simulink model "MARC_Hinf"  (R2016b)
settings: Solver=VariableStepAuto  StartTime=0.0  StopTime=150  RelTol=1e-3
values from neighbouring files (symbols this model uses):
  Aa = [zeros(n,n) Cp;zeros(np,n) Ap]    [g_MRAC_design_Hinf.m]
  Aref = Aa - Ba*KxT    [g_MRAC_design_Hinf.m]
  Ba = [Dp;Bp]    [g_MRAC_design_Hinf.m]
  Bref = [-eye(n);zeros(np,n)]    [g_MRAC_design_Hinf.m]
  Ca = [zeros(n,n) Cp]    [g_MRAC_design_Hinf.m]
  Cref = Ca    [g_MRAC_design_Hinf.m]
  DA = 0.75*eye(n)    [g_MRAC_design_Hinf.m]
  Gama_theta_ = eye(13)*5    [g_MRAC_design_Hinf.m]
  if_sat_modification = 1    [g_MRAC_design_Hinf.m]
  KxT = [KI KF]    [g_Hinf_design.m]
  Lv = Pv*inv(Rv)    [g_MRAC_design_Hinf.m]
  Pv = are(Aref',inv(Rv), Qv)    [g_MRAC_design_Hinf.m]
undefined symbols (not defined in the file): n, np
libraries: simulink x10
settings Model: Creator=user  LastModifiedBy=xiaoliang

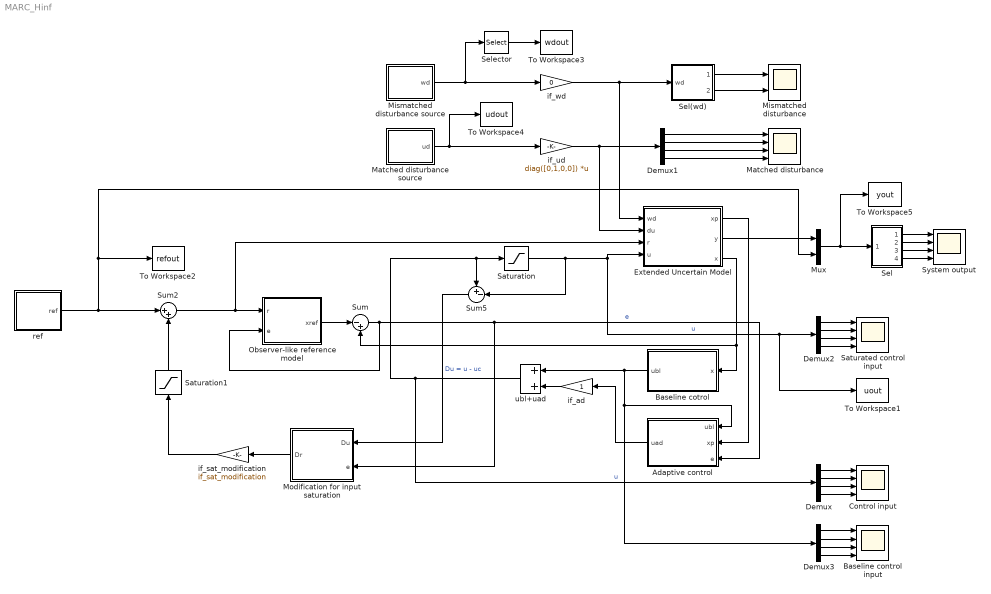
== system MARC_Hinf ==
  Adaptive control : Subsystem  mask{Gama_theta_=Gama_theta_, Pref=Pv, Ba=Ba, theta_max=[1 1 1 1.5]*1, es=[0.8 0.8 0.8 0.8]}
  Baseline control input : Scope  NumInputPorts=4
  Baseline cotrol : Subsystem  mask{KxT=KxT}
  Control input : Scope  NumInputPorts=4
  Demux{,1..3} (4 alike) : Demux
  Extended Uncertain Model : Subsystem  mask{Aa=Aa, Ba=Ba, Ca=Ca, Bref=Bref, Dex=[n+1:n+np], DA=DA, THETA0=rand(4,9)*0.5}
  Matched disturbance : Scope  NumInputPorts=4
  Matched disturbance source : Subsystem  mask{wb=0.2, k=0.5, Ts=0.001}
      mask prompts: wb "wb (Filter bandwidth)"; k "k (Signal standard deviation)"; Ts "Ts (Sample time)"
  Mismatched disturbance : Scope  NumInputPorts=2
  Mismatched disturbance source : Subsystem  mask{wb=2.5, k=0.4, Ts=0.001}
      mask prompts: wb "wb (Filter bandwidth)"; k "k (Signal standard deviation)"; Ts "Ts (Sample time)"
  Modification for input saturation : Subsystem  mask{Pv=Pv, Bref=Bref, Gama_du=-diag([1 1 1 1])*2}
  Mux : Mux  Inputs=2
  Observer-like reference model : Subsystem  mask{Aref=Aref, Bref=Bref, Cref=Cref, Lv=Lv}
  Saturated control input : Scope  NumInputPorts=4
  Saturation : Saturate  UpperLimit=inf  LowerLimit=-inf
  Saturation1 : Saturate  UpperLimit=1  LowerLimit=-1
  Sel : Subsystem
  Sel(wd) : Subsystem
  Selector : Selector  InputPortWidth=13  IndexOptions=Index vector (dialog)  Indices=[5:10]  OutputSizes=1
  Sum : Sum  Inputs=|-+
  Sum2 : Sum  Inputs=|++
  Sum5 : Sum  Inputs=+-|
  System output : Scope  NumInputPorts=4
  To Workspace1 : ToWorkspace  VariableName=uout  SaveFormat=Timeseries  SampleTime=-1
  To Workspace2 : ToWorkspace  VariableName=refout  SaveFormat=Timeseries  SampleTime=-1
  To Workspace3 : ToWorkspace  VariableName=wdout  SaveFormat=Timeseries  SampleTime=-1
  To Workspace4 : ToWorkspace  VariableName=udout  SaveFormat=Timeseries  SampleTime=-1
  To Workspace5 : ToWorkspace  VariableName=yout  SaveFormat=Timeseries  SampleTime=-1
  if_ad : Gain
  if_sat_modification : Gain  Gain=if_sat_modification
  if_ud : Gain  Gain=diag([0,1,0,0])  Multiplication=Matrix(K*u)
  if_wd : Gain  Gain=0
  ref : Subsystem
  ubl+uad : Sum
  wires:
  Mismatched disturbance source/1(wd) -> if_wd/1, Selector/1
  Extended Uncertain Model/3(x) -> Sum/2, Baseline cotrol/1(x)
  Extended Uncertain Model/1(xp) -> Adaptive control/2(xp)
  Observer-like reference model/1(xref) -> Sum/1
  Sum/1 -> Modification for input saturation/2(e), Adaptive control/3(e), Observer-like reference model/2(e)  "e"
  Adaptive control/1(uad) -> if_ad/1
  Baseline cotrol/1(ubl) -> Demux3/1, Adaptive control/1(ubl), ubl+uad/1
  Extended Uncertain Model/2(y) -> Mux/1
  Mux/1 -> Sel/1("[y;r]"), To Workspace5/1
  Sel/1(1) -> System output/1
  Sel/2(2) -> System output/2
  Sel/3(3) -> System output/3
  Sel/4(4) -> System output/4
  Matched disturbance source/1(ud) -> if_ud/1, To Workspace4/1
  ubl+uad/1 -> Saturation/1, Sum5/1, Demux/1  "u"
  Demux/1 -> Control input/1
  Demux/2 -> Control input/2
  Demux/3 -> Control input/3
  Demux/4 -> Control input/4
  if_wd/1 -> Extended Uncertain Model/1(wd), Sel(wd)/1(wd)
  if_ud/1 -> Demux1/1, Extended Uncertain Model/2(du)
  Demux1/1 -> Matched disturbance/1
  Demux1/2 -> Matched disturbance/2
  Demux1/3 -> Matched disturbance/3
  Demux1/4 -> Matched disturbance/4
  if_ad/1 -> ubl+uad/2
  Selector/1 -> To Workspace3/1
  Demux2/1 -> Saturated control input/1
  Demux2/2 -> Saturated control input/2
  Demux2/3 -> Saturated control input/3
  Demux2/4 -> Saturated control input/4
  Saturation/1 -> Sum5/2, To Workspace1/1, Demux2/1, Extended Uncertain Model/4(u)  "u"
  Sum2/1 -> Extended Uncertain Model/3(r), Observer-like reference model/1(r)
  ref/1(ref) -> Mux/2, To Workspace2/1, Sum2/1
  Modification for input saturation/1(Dr) -> if_sat_modification/1
  Sum5/1 -> Modification for input saturation/1(Du)  "Du = u - uc"
  if_sat_modification/1 -> Saturation1/1
  Sel(wd)/1(wd(1,2,3)) -> Mismatched disturbance/1
  Sel(wd)/2(wd(4,5,6)) -> Mismatched disturbance/2
  Saturation1/1 -> Sum2/2
  Demux3/1 -> Baseline control input/1
  Demux3/2 -> Baseline control input/2
  Demux3/3 -> Baseline control input/3
  Demux3/4 -> Baseline control input/4

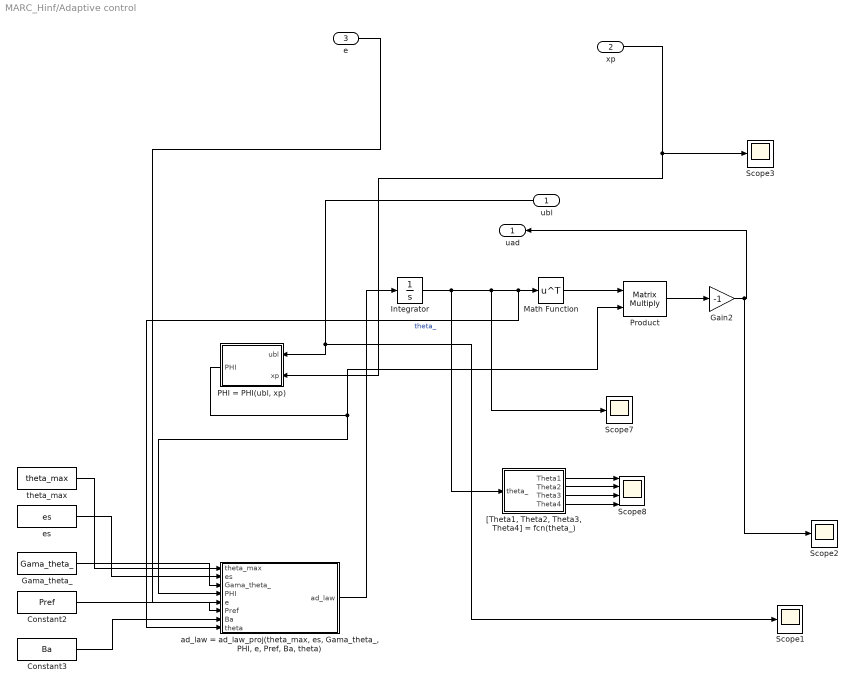
== system MARC_Hinf/Adaptive control ==
  ubl : Inport
  xp : Inport  Port=2
  e : Inport  Port=3
  Constant2 : Constant  Value=Pref
  Constant3 : Constant  Value=Ba
  Gain2 : Gain  Gain=-1
  Gama_theta_ : Constant  Value=Gama_theta_
  Integrator : Integrator  UpperSaturationLimit=4  LowerSaturationLimit=-4  IgnoreLimit=on
  Math Function : Math  Operator=transpose  SaturateOnIntegerOverflow=on
  "PHI = PHI(ubl, xp)" : MATLAB Function  TreatAsAtomicUnit=on
  Product : Product  Multiplication=Matrix(*)
  Scope{1..3,7} (4 alike) : Scope
  Scope8 : Scope  NumInputPorts=4
  "[Theta1, Theta2, Theta3, Theta4] = fcn(theta_)" : MATLAB Function  TreatAsAtomicUnit=on
  "ad_law = ad_law_proj(theta_max, es, Gama_theta_, PHI, e, Pref, Ba, theta)" : MATLAB Function  TreatAsAtomicUnit=on
  es : Constant  Value=es
  theta_max : Constant  Value=theta_max
  uad : Outport
  wires:
  Constant2/1 -> "ad_law = ad_law_proj(theta_max, es, Gama_theta_, PHI, e, Pref, Ba, theta)"/6(Pref)
  "[Theta1, Theta2, Theta3, Theta4] = fcn(theta_)"/1(Theta1) -> Scope8/1
  "[Theta1, Theta2, Theta3, Theta4] = fcn(theta_)"/2(Theta2) -> Scope8/2
  Gain2/1 -> Scope2/1, uad/1
  Integrator/1 -> "[Theta1, Theta2, Theta3, Theta4] = fcn(theta_)"/1(theta_), Scope7/1, "ad_law = ad_law_proj(theta_max, es, Gama_theta_, PHI, e, Pref, Ba, theta)"/8(theta), Math Function/1  "theta_"
  Math Function/1 -> Product/1
  Product/1 -> Gain2/1
  "ad_law = ad_law_proj(theta_max, es, Gama_theta_, PHI, e, Pref, Ba, theta)"/1(ad_law) -> Integrator/1
  Gama_theta_/1 -> "ad_law = ad_law_proj(theta_max, es, Gama_theta_, PHI, e, Pref, Ba, theta)"/3(Gama_theta_)
  e/1 -> "ad_law = ad_law_proj(theta_max, es, Gama_theta_, PHI, e, Pref, Ba, theta)"/5(e)
  "PHI = PHI(ubl, xp)"/1(PHI) -> "ad_law = ad_law_proj(theta_max, es, Gama_theta_, PHI, e, Pref, Ba, theta)"/4(PHI), Product/2
  Constant3/1 -> "ad_law = ad_law_proj(theta_max, es, Gama_theta_, PHI, e, Pref, Ba, theta)"/7(Ba)
  xp/1 -> Scope3/1, "PHI = PHI(ubl, xp)"/2(xp)
  ubl/1 -> Scope1/1, "PHI = PHI(ubl, xp)"/1(ubl)
  es/1 -> "ad_law = ad_law_proj(theta_max, es, Gama_theta_, PHI, e, Pref, Ba, theta)"/2(es)
  theta_max/1 -> "ad_law = ad_law_proj(theta_max, es, Gama_theta_, PHI, e, Pref, Ba, theta)"/1(theta_max)
  "[Theta1, Theta2, Theta3, Theta4] = fcn(theta_)"/3(Theta3) -> Scope8/3
  "[Theta1, Theta2, Theta3, Theta4] = fcn(theta_)"/4(Theta4) -> Scope8/4

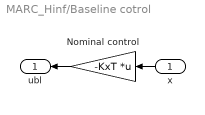
== system MARC_Hinf/Baseline cotrol ==
  x : Inport
  Nominal control : Gain  Gain=-KxT  Multiplication=Matrix(K*u)
  ubl : Outport
  wires:
  Nominal control/1 -> ubl/1
  x/1 -> Nominal control/1

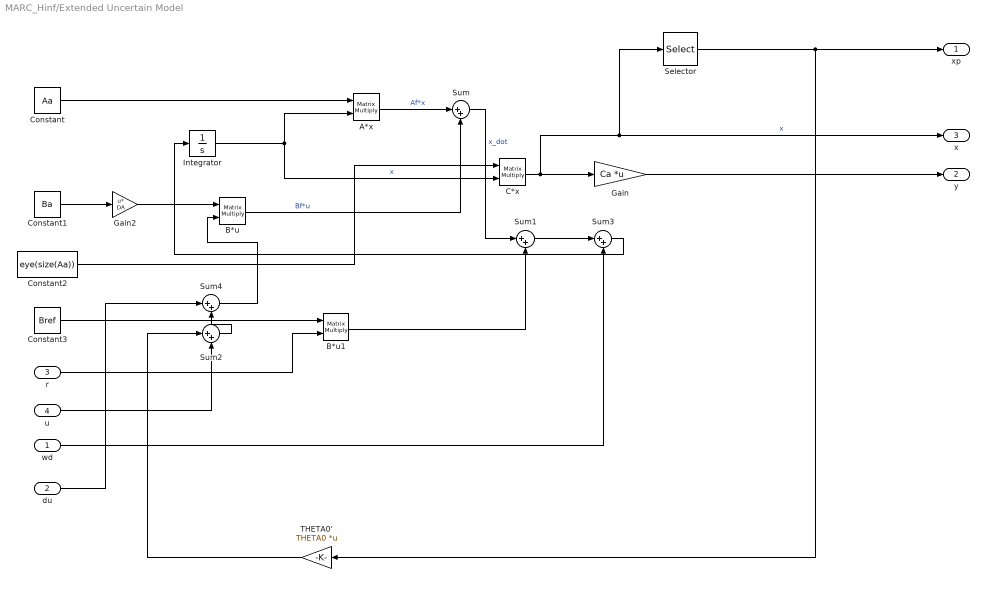
== system MARC_Hinf/Extended Uncertain Model ==
  wd : Inport
  du : Inport  Port=2
  r : Inport  Port=3
  u : Inport  Port=4
  A*x : Product  Multiplication=Matrix(*)
  B*u : Product  Multiplication=Matrix(*)
  B*u1 : Product  Multiplication=Matrix(*)
  C*x : Product  Multiplication=Matrix(*)
  Constant : Constant  Value=Aa
  Constant1 : Constant  Value=Ba
  Constant2 : Constant  Value=eye(size(Aa))
  Constant3 : Constant  Value=Bref
  Gain : Gain  Gain=Ca  Multiplication=Matrix(K*u)
  Gain2 : Gain  Gain=DA  Multiplication=Matrix(u*K)
  Integrator : Integrator  UpperSaturationLimit=1000  LowerSaturationLimit=-1000
  Selector : Selector  InputPortWidth=size(Aa,1)  IndexOptions=Index vector (dialog)  Indices=Dex  OutputSizes=1
  Sum{,1..4} (5 alike) : Sum  Inputs=|++
  THETA0' : Gain  Gain=THETA0  Multiplication=Matrix(K*u)
  xp : Outport
  y : Outport  Port=2
  x : Outport  Port=3
  wires:
  B*u/1 -> Sum/2  "Bf*u"
  Constant/1 -> A*x/1
  Integrator/1 -> A*x/2, C*x/2  "x"
  Constant1/1 -> Gain2/1
  Constant2/1 -> C*x/1
  A*x/1 -> Sum/1  "Af*x"
  C*x/1 -> x/1, Selector/1, Gain/1  "x"
  Gain/1 -> y/1
  r/1 -> B*u1/2
  B*u1/1 -> Sum1/2
  Sum/1 -> Sum1/1  "x_dot"
  Selector/1 -> THETA0'/1, xp/1
  Constant3/1 -> B*u1/1
  Gain2/1 -> B*u/1
  Sum1/1 -> Sum3/1
  wd/1 -> Sum3/2
  Sum3/1 -> Integrator/1
  u/1 -> Sum2/2
  THETA0'/1 -> Sum2/1
  Sum2/1 -> Sum4/2
  du/1 -> Sum4/1
  Sum4/1 -> B*u/2

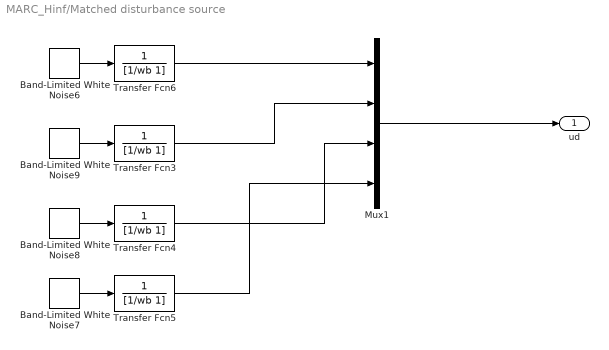
== system MARC_Hinf/Matched disturbance source ==
  Band-Limited White Noise6 : simulink/Sources/Band-Limited White Noise  Cov=2*k^2/wb  Ts=Ts  seed=[23314]
  Band-Limited White Noise7 : simulink/Sources/Band-Limited White Noise  Cov=2*k^2/wb  Ts=Ts  seed=[23313]
  Band-Limited White Noise8 : simulink/Sources/Band-Limited White Noise  Cov=2*k^2/wb  Ts=Ts  seed=[23312]
  Band-Limited White Noise9 : simulink/Sources/Band-Limited White Noise  Cov=2*k^2/wb  Ts=Ts  seed=[23311]
  Mux1 : Mux
  Transfer Fcn{3..6} (4 alike) : TransferFcn  Denominator=[1/wb 1]
  ud : Outport
  wires:
  Band-Limited White Noise7/1 -> Transfer Fcn5/1
  Band-Limited White Noise6/1 -> Transfer Fcn6/1
  Band-Limited White Noise8/1 -> Transfer Fcn4/1
  Band-Limited White Noise9/1 -> Transfer Fcn3/1
  Transfer Fcn3/1 -> Mux1/2
  Transfer Fcn6/1 -> Mux1/1
  Mux1/1 -> ud/1
  Transfer Fcn4/1 -> Mux1/3
  Transfer Fcn5/1 -> Mux1/4

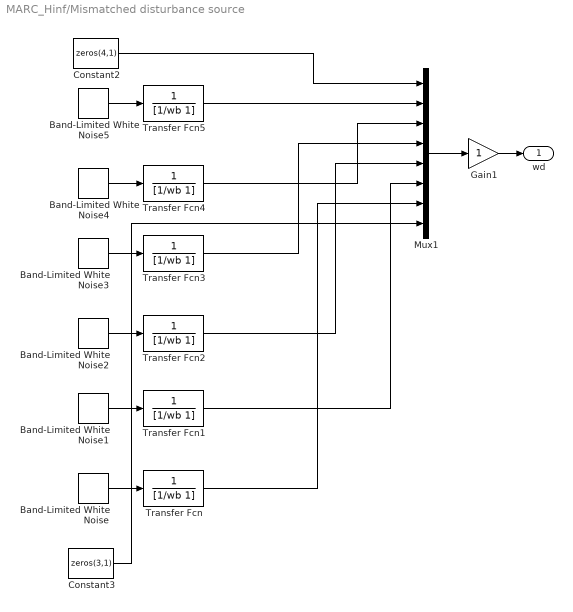
== system MARC_Hinf/Mismatched disturbance source ==
  Band-Limited White Noise : simulink/Sources/Band-Limited White Noise  Cov=2*k^2/wb  Ts=Ts  seed=[23345]
  Band-Limited White Noise1 : simulink/Sources/Band-Limited White Noise  Cov=2*k^2/wb  Ts=Ts  seed=[23344]
  Band-Limited White Noise2 : simulink/Sources/Band-Limited White Noise  Cov=2*k^2/wb  Ts=Ts  seed=[23341]
  Band-Limited White Noise3 : simulink/Sources/Band-Limited White Noise  Cov=2*k^2/wb  Ts=Ts  seed=[23340]
  Band-Limited White Noise4 : simulink/Sources/Band-Limited White Noise  Cov=2*k^2/wb  Ts=Ts  seed=[23343]
  Band-Limited White Noise5 : simulink/Sources/Band-Limited White Noise  Cov=2*k^2/wb  Ts=Ts  seed=[23342]
  Constant2 : Constant  Value=zeros(4,1)
  Constant3 : Constant  Value=zeros(3,1)
  Gain1 : Gain
  Mux1 : Mux  Inputs=8
  Transfer Fcn{,1..5} (6 alike) : TransferFcn  Denominator=[1/wb 1]
  wd : Outport
  wires:
  Transfer Fcn3/1 -> Mux1/4
  Mux1/1 -> Gain1/1
  Band-Limited White Noise3/1 -> Transfer Fcn3/1
  Band-Limited White Noise2/1 -> Transfer Fcn2/1
  Band-Limited White Noise1/1 -> Transfer Fcn1/1
  Transfer Fcn4/1 -> Mux1/3
  Transfer Fcn1/1 -> Mux1/6
  Transfer Fcn5/1 -> Mux1/2
  Transfer Fcn2/1 -> Mux1/5
  Transfer Fcn/1 -> Mux1/7
  Band-Limited White Noise/1 -> Transfer Fcn/1
  Band-Limited White Noise4/1 -> Transfer Fcn4/1
  Band-Limited White Noise5/1 -> Transfer Fcn5/1
  Gain1/1 -> wd/1
  Constant2/1 -> Mux1/1
  Constant3/1 -> Mux1/8

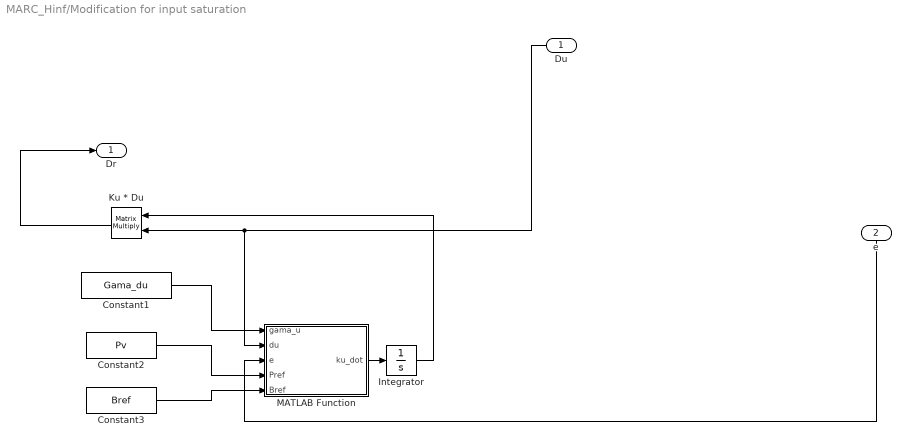
== system MARC_Hinf/Modification for input saturation ==
  Du : Inport
  e : Inport  Port=2
  Constant1 : Constant  Value=Gama_du
  Constant2 : Constant  Value=Pv
  Constant3 : Constant  Value=Bref
  Integrator : Integrator
  Ku * Du : Product  Multiplication=Matrix(*)
  MATLAB Function : MATLAB Function  TreatAsAtomicUnit=on
  Dr : Outport
  wires:
  Ku * Du/1 -> Dr/1
  e/1 -> MATLAB Function/3(e)
  Du/1 -> MATLAB Function/2(du), Ku * Du/2
  Constant1/1 -> MATLAB Function/1(gama_u)
  Integrator/1 -> Ku * Du/1
  Constant3/1 -> MATLAB Function/5(Bref)
  Constant2/1 -> MATLAB Function/4(Pref)
  MATLAB Function/1(ku_dot) -> Integrator/1

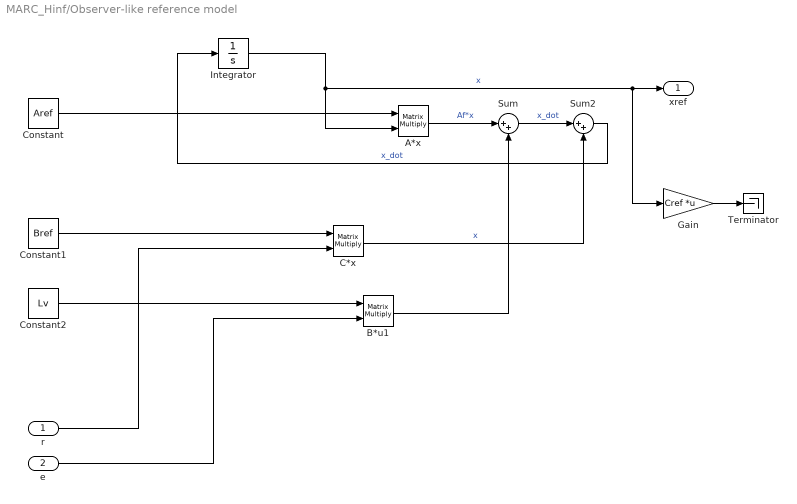
== system MARC_Hinf/Observer-like reference model ==
  r : Inport
  e : Inport  Port=2
  A*x : Product  Multiplication=Matrix(*)
  B*u1 : Product  Multiplication=Matrix(*)
  C*x : Product  Multiplication=Matrix(*)
  Constant : Constant  Value=Aref
  Constant1 : Constant  Value=Bref
  Constant2 : Constant  Value=Lv
  Gain : Gain  Gain=Cref  Multiplication=Matrix(K*u)
  Integrator : Integrator  UpperSaturationLimit=1000  LowerSaturationLimit=-1000
  Sum : Sum  Inputs=|++
  Sum2 : Sum  Inputs=|++
  Terminator : Terminator
  xref : Outport
  wires:
  A*x/1 -> Sum/1  "Af*x"
  C*x/1 -> Sum2/2  "x"
  Integrator/1 -> xref/1, Gain/1, A*x/2  "x"
  Sum2/1 -> Integrator/1  "x_dot"
  Constant/1 -> A*x/1
  Constant2/1 -> B*u1/1
  e/1 -> B*u1/2
  B*u1/1 -> Sum/2
  Sum/1 -> Sum2/1  "x_dot"
  Constant1/1 -> C*x/1
  r/1 -> C*x/2
  Gain/1 -> Terminator/1

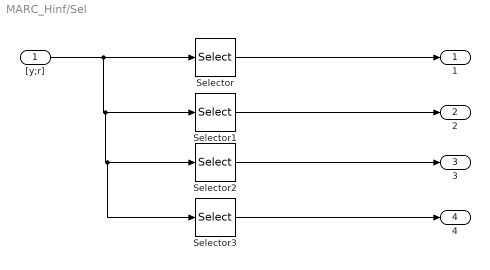
== system MARC_Hinf/Sel ==
  "[y;r]" : Inport
  Selector : Selector  InputPortWidth=8  IndexOptions=Index vector (dialog)  Indices=[1 5]  OutputSizes=1
  Selector1 : Selector  InputPortWidth=8  IndexOptions=Index vector (dialog)  Indices=[2 6]  OutputSizes=1
  Selector2 : Selector  InputPortWidth=8  IndexOptions=Index vector (dialog)  Indices=[3 7]  OutputSizes=1
  Selector3 : Selector  InputPortWidth=8  IndexOptions=Index vector (dialog)  Indices=[4 8]  OutputSizes=1
  1 : Outport
  2 : Outport  Port=2
  3 : Outport  Port=3
  4 : Outport  Port=4
  wires:
  Selector1/1 -> 2/1
  Selector/1 -> 1/1
  Selector2/1 -> 3/1
  Selector3/1 -> 4/1
  "[y;r]"/1 -> Selector3/1, Selector2/1, Selector1/1, Selector/1

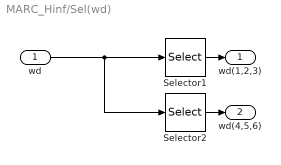
== system MARC_Hinf/Sel(wd) ==
  wd : Inport
  Selector1 : Selector  InputPortWidth=13  IndexOptions=Index vector (dialog)  Indices=[5 6 7]  OutputSizes=1
  Selector2 : Selector  InputPortWidth=13  IndexOptions=Index vector (dialog)  Indices=[8 9 10]  OutputSizes=1
  wd(1,2,3) : Outport
  wd(4,5,6) : Outport  Port=2
  wires:
  wd/1 -> Selector2/1, Selector1/1
  Selector2/1 -> wd(4,5,6)/1
  Selector1/1 -> wd(1,2,3)/1

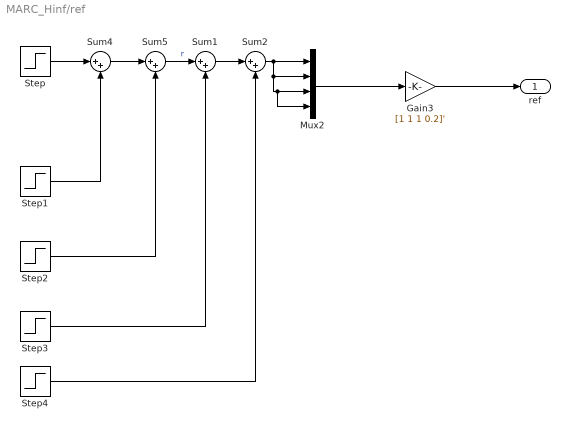
== system MARC_Hinf/ref ==
  Gain3 : Gain  Gain=[1 1 1 0.2]'
  Mux2 : Mux
  Step : Step  SampleTime=0
  Step1 : Step  Time=20  After=-2  SampleTime=0.001
  Step2 : Step  Time=40  SampleTime=0.001
  Step3 : Step  Time=60  After=1.0  SampleTime=0.001
  Step4 : Step  Time=80  After=-1.0  SampleTime=0.001
  Sum{1..2,4..5} (4 alike) : Sum  Inputs=|++
  ref : Outport
  wires:
  Mux2/1 -> Gain3/1
  Step/1 -> Sum4/1
  Step1/1 -> Sum4/2
  Step2/1 -> Sum5/2
  Sum4/1 -> Sum5/1
  Gain3/1 -> ref/1
  Sum5/1 -> Sum1/1  "r"
  Step3/1 -> Sum1/2
  Sum1/1 -> Sum2/1
  Step4/1 -> Sum2/2
  Sum2/1 -> Mux2/4, Mux2/3, Mux2/2, Mux2/1

== matlab function MARC_Hinf/Adaptive control/[Theta1, Theta2, Theta3, Theta4] = fcn(theta_) ==
  data: theta_ input; Theta1 output; Theta2 output; Theta3 output; Theta4 output
function  [Theta1, Theta2, Theta3, Theta4] = fcn(theta_)
%#codegen
Theta1 = norm(theta_(:,1));
Theta2 = norm(theta_(:,2));
Theta3 = norm(theta_(:,3));
Theta4 = norm(theta_(:,4));

== matlab function MARC_Hinf/Adaptive control/PHI = PHI(ubl, xp) ==
  data: ubl input; PHI output; xp input
function PHI = PHI(ubl, xp)
%#codegen
PHI = [ubl' xp']';

== matlab function MARC_Hinf/Modification for input saturation/MATLAB Function ==
  data: gama_u input; ku_dot output; du input; e input; Pref input; Bref input
function ku_dot = fcn(gama_u,du,e,Pref,Bref)
%#codegen

ku_dot = gama_u*du*e'*Pref*Bref;

== matlab function MARC_Hinf/Adaptive control/ad_law = ad_law_proj(theta_max, es, Gama_theta_, PHI, e, Pref, Ba, theta) ==
  data: theta_max input; es input; Gama_theta_ input; ad_law output; PHI input; e input; Pref input; Ba input; theta input
function ad_law = ad_law_proj(theta_max, es, Gama_theta_, PHI, e, Pref, Ba, theta)
% theta_max = [0.5 3.5];
% es = [0.1 0.1];
% ad_law = Gama_theta_*PHI*e'*Pref*Ba;
m = size(Gama_theta_,1);
n = size(Ba, 2);
% Gama_theta = Gama_theta_(n+1:m,n+1:m);
ad_law = zeros(m, n);
ad_law0 = PHI*e'*Pref*Ba;
for i = 1:n
    fi = f_convex(theta(:,i),theta_max(i),es(i));
    Dfi = Df(theta(:,i), theta_max(i), es(i));
    if  fi > 0 && ad_law0(:,i)'* Gama_theta_ * Dfi > 0
        Df_theta2 = norm(Dfi'* Gama_theta_ * Dfi);
        ad_law(:,i) = Gama_theta_ * (ad_law0(:,i) - Dfi * Dfi'/Df_theta2 * Gama_theta_ * ad_law0(:,i) *fi);
    else
        ad_law(:,i)= Gama_theta_ * ad_law0(:,i);
    end
end
sig = 0.1;
ad_law = ad_law - Gama_theta_*sig*norm(e'*Pref*Ba)*theta;
function fi = f_convex(u, umax, es)
fi = ((1+es)*(norm(u))^2 - umax^2)/(es*umax^2);


function Dfi = Df(u, umax, es)
Dfi = 2*(1+es)/(es*umax)*u;
